simulink model "SimulinkTP7"  (R2018b)
settings: Solver=VariableStepAuto  StartTime=0.0  StopTime=0.003  RelTol=1e-3
libraries: fl_lib x12, nesl_utility x7, elec_lib x2
settings Model: Creator=A47521  LastModifiedBy=A47521

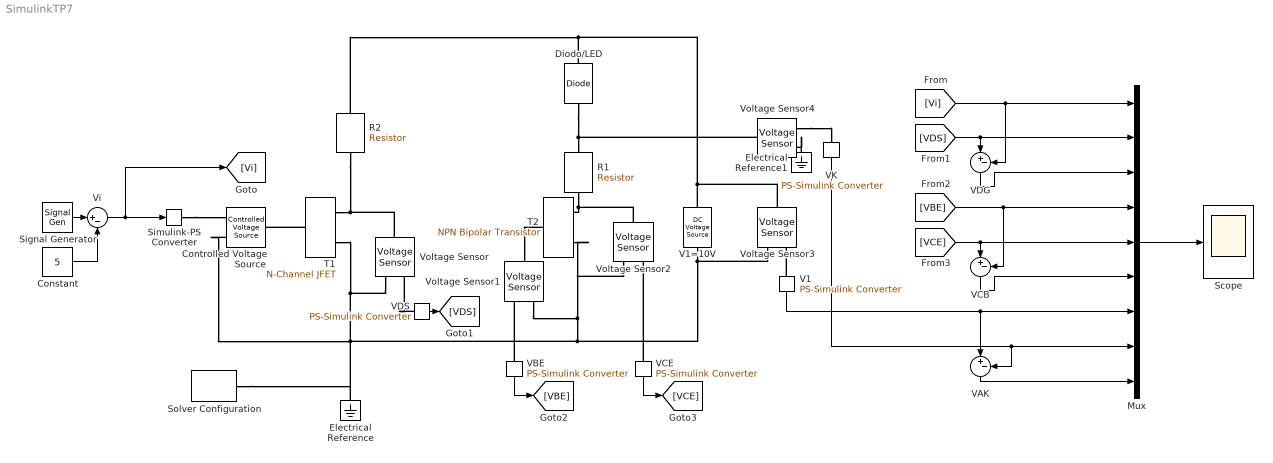
== system SimulinkTP7 ==
  Constant : Constant  Value=5
  Controlled Voltage Source : fl_lib/Electrical/Electrical Sources/Controlled Voltage Source
  Diodo/LED : fl_lib/Electrical/Electrical Elements/Diode  Vf=3 V  Ron=0.3 Ohm  Goff=1e-8 1/Ohm  i_specify=off  i_priority=None  i=0 A  i_nominal_specify=off  i_nominal_unit=A  i_nominal_value=1  v_specify=off  v_priority=None  v=0 V  v_nominal_specify=off  v_nominal_unit=V  v_nominal_value=1
  Electrical Reference : fl_lib/Electrical/Electrical Elements/Electrical Reference
  Electrical Reference1 : fl_lib/Electrical/Electrical Elements/Electrical Reference
  Mux : Mux  Inputs=9
  R1 : fl_lib/Electrical/Electrical Elements/Resistor  R=100 Ohm  i_specify=off  i_priority=None  i=0 A  i_nominal_specify=off  i_nominal_unit=A  i_nominal_value=1  v_specify=off  v_priority=None  v=0 V  v_nominal_specify=off  v_nominal_unit=V  v_nominal_value=1
  R2 : fl_lib/Electrical/Electrical Elements/Resistor  R=47 kOhm  i_specify=off  i_priority=None  i=0 A  i_nominal_specify=off  i_nominal_unit=A  i_nominal_value=1  v_specify=off  v_priority=None  v=0 V  v_nominal_specify=off  v_nominal_unit=V  v_nominal_value=1
  Scope : Scope
  Signal Generator : SignalGenerator  WaveForm=square  Amplitude=5  Frequency=1000
  Simulink-PS Converter : nesl_utility/Simulink-PS Converter  PhysicalDomain=network_engine_domain  SubClassName=ps_input  LeftPortType=input  RightPortType=output  PseudoPeriodic=off  Frequencies=[]  NoiseDistribution=none  NoiseParameters=[]  Unit=1  AffineConversion=off  FilteringAndDerivatives=provide  SimscapeFilterOrder=1  InputFilterTimeConstant=0.001  UdotUserProvided=0
  Solver Configuration : nesl_utility/Solver Configuration  PhysicalDomain=network_engine_domain  SubClassName=solver  LeftPortType=input  RightPortType=generic  Tones=[]  Harmonics=[]  SimulateNoise=off  Profile=off  UseLocalSampling=off  EnableSwitchedLinearOptims=on  FrequencyDomain=off  UseCCode=off  RelTol=0.001  AbsTol=1e-06  MinStep=1e-09  ToWorkspace=off  RevertToSquareIcSolve=off  NumHomotopyIterations=100  PhasorMode=off  PhasorModeNumHarmonics=1  DoDC=off  ResidualTolerance=1e-09  UseLocalSolver=off  LocalSolverChoice=NE_BACKWARD_EULER_ADVANCER  LocalSolverSampleTime=0.001  DoFixedCost=off  MaxNonlinIter=3  MaxModeIter=2  LinearAlgebra=auto  EquationFormulation=NE_TIME_EF  DelaysMemoryBudget=1024  AutomaticFiltering=on  FilteringTimeConstant=0.001  PartitionStorageMethod=AS_NEEDED  PartitionMemoryBudget=1024
  T1 : elec_lib/Semiconductor Devices/N-Channel JFET  parameterization=1  prmDatasheet=1  prmEquCoeff=1  Igss=-1 nA  Idss=12 mA  Idss_v=[ 0 15 ] V  ssig=[ 3e+3 10 ] uS  ssig_v=[ 0 15 ] V  Beta=6.2e-4 A/V^2  IS=5e-10 A  Vt0=-2.3 V  Lchannel=0.003 1/V  Tmeas=25 degC  RS=1e-4 Ohm  RD=0.01 Ohm  C_param=1  C_GS=3 pF  C_GD=1.5 pF  C_iss=4.5 pF  C_rss=1.5 pF  Igss_T2=-200 nA  EG=1.11 eV  XTI=3  dVt0_dT=-2 mV/K  Idss_T2=2.5 mA  Tmeas2=125 degC  BEXDatasheet=-1.5  BEXEquCoeff=-1.5  TdeviceDatasheet=25 degC  TdeviceEquCoeff=25 degC  Rth=[ 0 10 ] K/W  thermal_mass_parameterization=1  thermal_mass=[ 0 1 ] J/K  thermal_time_constant=[ 0 10 ] s  thermal_mass_initial_temperatures=[ 25 25 ] degC
      settings: SourceProductName=Simscape Electronics  SourceProductBaseCode=SN
  T2 : elec_lib/Semiconductor Devices/NPN Bipolar Transistor  parameterization=1  prmDatasheet=1  prmEquCoeff=1  BF=100  IS=1e-14 A  ec=1  VAF=200 V  hfe=100  hoe=5e-5 1/Ohm  Ic_h=1 mA  Vce_h=5 V  V1=0.55 V  I1=0.5 mA  BR=1  Tmeas=25 degC  RC=0.01 Ohm  RE=1e-4 Ohm  RB=1 Ohm  C_BC=5 pF  C_BE=5 pF  TF=0 us  TR=0 us  hfe_T2=125  XTB=0  V1_T2=0.45 V  I1_T2=0.5 mA  Tmeas2=125 degC  EG=1.11 eV  XTI=3  TdeviceDatasheet=25 degC  TdeviceEquCoeff=25 degC  Rth=[ 0 10 ] K/W  thermal_mass_parameterization=1  thermal_mass=[ 0 1 ] J/K  thermal_time_constant=[ 0 10 ] s  thermal_mass_initial_temperatures=[ 25 25 ] degC
      settings: SourceProductName=Simscape Electronics  SourceProductBaseCode=SN
  V1 : nesl_utility/PS-Simulink Converter  PhysicalDomain=network_engine_domain  SubClassName=ps_output  LeftPortType=input  RightPortType=output  PseudoPeriodic=off  Frequencies=[]  Unit=1  AffineConversion=off
  V1=10V : fl_lib/Electrical/Electrical Sources/DC Voltage Source  v0=10 V
  VAK : Sum  Inputs=|+-
  VBE : nesl_utility/PS-Simulink Converter  PhysicalDomain=network_engine_domain  SubClassName=ps_output  LeftPortType=input  RightPortType=output  PseudoPeriodic=off  Frequencies=[]  Unit=1  AffineConversion=off
  VCB : Sum  Inputs=|+-
  VCE : nesl_utility/PS-Simulink Converter  PhysicalDomain=network_engine_domain  SubClassName=ps_output  LeftPortType=input  RightPortType=output  PseudoPeriodic=off  Frequencies=[]  Unit=1  AffineConversion=off
  VDG : Sum  Inputs=|+-
  VDS : nesl_utility/PS-Simulink Converter  PhysicalDomain=network_engine_domain  SubClassName=ps_output  LeftPortType=input  RightPortType=output  PseudoPeriodic=off  Frequencies=[]  Unit=1  AffineConversion=off
  VK : nesl_utility/PS-Simulink Converter  PhysicalDomain=network_engine_domain  SubClassName=ps_output  LeftPortType=input  RightPortType=output  PseudoPeriodic=off  Frequencies=[]  Unit=1  AffineConversion=off
  Vi : Sum  Inputs=|+-
  Voltage Sensor{,1..4} (5 alike) : fl_lib/Electrical/Electrical Sensors/Voltage Sensor
  wires:
  Signal Generator/1 -> Vi/1
  Vi/1 -> [Vi], Simulink-PS Converter/1
  Constant/1 -> Vi/2
  VDS/1 -> [VDS]
  VBE/1 -> [VBE]
  VCE/1 -> [VCE]
  Mux/1 -> Scope/1
  [Vi] -> Mux/1, VDG/2
  [VDS] -> VDG/1, Mux/2
  VDG/1 -> Mux/3
  [VBE] -> Mux/4, VCB/2
  [VCE] -> VCB/1, Mux/5
  VCB/1 -> Mux/6
  V1/1 -> VAK/1, Mux/7
  VK/1 -> VAK/2, Mux/8
  VAK/1 -> Mux/9
  connections:
  R1/RConn1 -- Voltage Sensor2/LConn1 -- T2/RConn1
  Diodo/LED/RConn1 -- Voltage Sensor4/LConn1 -- R1/LConn1
  V1=10V/LConn1 -- Voltage Sensor3/LConn1 -- Diodo/LED/LConn1 -- R2/LConn1
  R2/RConn1 -- Voltage Sensor/LConn1 -- T1/RConn1
  V1=10V/RConn1 -- Voltage Sensor3/RConn2 -- T2/RConn2 -- Voltage Sensor2/RConn2 -- Voltage Sensor1/RConn2 -- Controlled Voltage Source/RConn2 -- Solver Configuration/RConn1 -- Electrical Reference/LConn1 -- T1/RConn2 -- Voltage Sensor/RConn2
  T1/LConn1 -- Controlled Voltage Source/LConn1
  Simulink-PS Converter/RConn1 -- Controlled Voltage Source/RConn1
  VDS/LConn1 -- Voltage Sensor/RConn1
  VBE/LConn1 -- Voltage Sensor1/RConn1
  VCE/LConn1 -- Voltage Sensor2/RConn1
  T2/LConn1 -- Voltage Sensor1/LConn1
  V1/LConn1 -- Voltage Sensor3/RConn1
  Electrical Reference1/LConn1 -- Voltage Sensor4/RConn2
  Voltage Sensor4/RConn1 -- VK/LConn1
